simulink model "create_weather_data"  (Simulink 8.1)
settings: Solver=FixedStepDiscrete  StartTime=0.0  StopTime=31*24*3600  FixedStep=600  RelTol=1e-3
settings Model: Creator=sfrank1  LastModifiedBy=sfrank1
settings DataIOCC: SignalLoggingSaveFormat=Dataset
settings OptimizationCC: ExpressionDepthLimit=128
settings DebuggingCC: FcnCallInpInsideContextMsg=EnableAllAsError
settings GRTTargetCC: CombineOutputUpdateFcns=on  GRTInterface=off

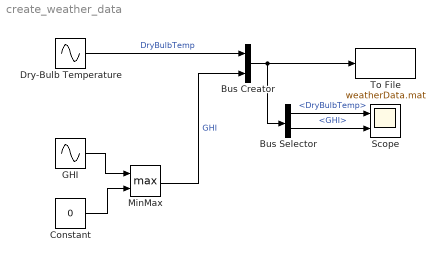
== system create_weather_data ==
  Bus Creator : BusCreator  Inputs='DryBulbTemp','GHI'
  Bus Selector : BusSelector  OutputSignals=DryBulbTemp,GHI
  Constant : Constant  Value=0
  Dry-Bulb Temperature : Sin  Amplitude=10  Bias=25  Frequency=(2*pi)/(60*60*24)  Phase=pi  SampleTime=0
  GHI : Sin  Amplitude=850  Bias=-100  Frequency=(2*pi)/(60*60*24)  Phase=-pi/2  SampleTime=0
  MinMax : MinMax  Function=max  Inputs=2
  Scope : Scope  NumInputPorts=2
      settings: YMin=-5~-5  YMax=5~5
  To File : ToFile  Filename=weatherData.mat  SaveFormat=Timeseries
  wires:
  GHI/1 -> MinMax/1
  Constant/1 -> MinMax/2
  MinMax/1 -> Bus Creator/2  "GHI"
  Dry-Bulb Temperature/1 -> Bus Creator/1  "DryBulbTemp"
  Bus Creator/1 -> Bus Selector/1, To File/1
  Bus Selector/1 -> Scope/1  "<DryBulbTemp>"
  Bus Selector/2 -> Scope/2  "<GHI>"
